simulink model "simulink_pre1"  (R2018a)
settings: Solver=VariableStepAuto  StartTime=0.0  StopTime=40  RelTol=1e-3
libraries: simulink x1
settings Model: Creator=bssho  LastModifiedBy=bssho

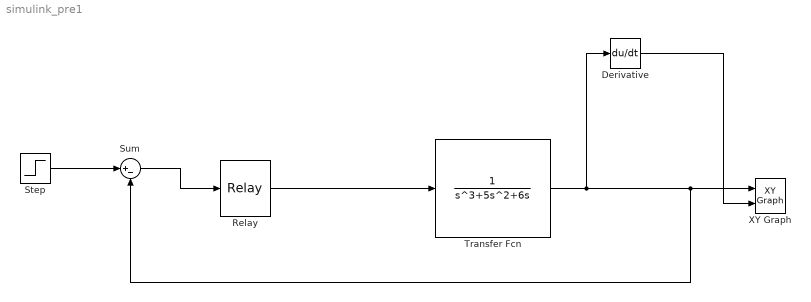
== system simulink_pre1 ==
  Derivative : Derivative
  Relay : Relay  OffOutputValue=-1
  Step : Step  SampleTime=0
  Sum : Sum  Inputs=|+-
  Transfer Fcn : TransferFcn  Denominator=[1 5 6 0]
  XY Graph : simulink/Sinks/XY Graph  xmin=-2  xmax=2  ymin=-1  ymax=1  st=-1
  wires:
  Relay/1 -> Transfer Fcn/1
  Transfer Fcn/1 -> Derivative/1, XY Graph/1, Sum/2
  Sum/1 -> Relay/1
  Step/1 -> Sum/1
  Derivative/1 -> XY Graph/2
